simulink model "test5"  (R2015a)
settings: Solver=ode45  StartTime=0.0  StopTime=20  RelTol=1e-3
InitFcn:
  | %% DSPBuilder Start
  | alt_dspbuilder_update_model(bdroot)
  | %% DSPBuilder End
libraries: allblocks_alteradspbuilder2 x10
settings Model: Creator=ASUS  LastModifiedBy=ASUS

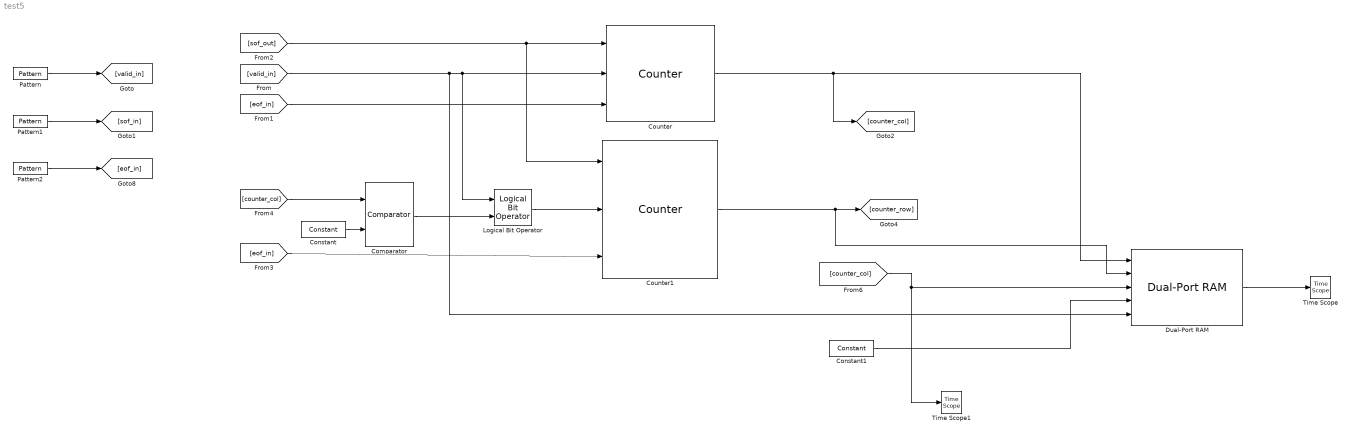
== system test5 ==
  Comparator : allblocks_alteradspbuilder2/Comparator  direction=a == b  pipeline_display=0  allowFloatingPointOverride=on  logOutputs=off  logFile=C:\Users\ASUS\Desktop\sift_fpga_final\Octave_2\tb_test5\test5_Comparator.fixedpointlog
  Constant : allblocks_alteradspbuilder2/Constant  mask_cst=3  BusType=Unsigned Integer  bwl=3  bwr=0  roundMode=Truncate  satMode=Wrap  SpecifyClock=off  allowFloatingPointOverride=on  logOutputs=off  logFile=C:\Users\ASUS\Desktop\sift_fpga_final\Octave_2\tb_test5\test5_Constant.fixedpointlog
  Constant1 : allblocks_alteradspbuilder2/Constant  mask_cst=1  BusType=Unsigned Integer  bwl=1  bwr=0  roundMode=Truncate  satMode=Wrap  SpecifyClock=off  allowFloatingPointOverride=on  logOutputs=off  logFile=C:\Users\ASUS\Desktop\sift_fpga_final\Octave_2\tb_test5\test5_Constant1.fixedpointlog
  Counter : allblocks_alteradspbuilder2/Counter  BusType=Unsigned Integer  bwl=5  bwr=0  use_modulo=on  modulo=4  SpecifyClock=off  direction=Increment  use_sload=off  use_sset=on  svalue=1  use_clk_ena=off  use_ena=on  use_sclr=on  pipeline_display=1
  Counter1 : allblocks_alteradspbuilder2/Counter  BusType=Unsigned Integer  bwl=5  bwr=0  use_modulo=on  modulo=4  SpecifyClock=off  direction=Increment  use_sload=off  use_sset=on  svalue=0  use_clk_ena=off  use_ena=on  use_sclr=on  pipeline_display=1
  Dual-Port RAM : allblocks_alteradspbuilder2/Dual-Port RAM  numwords=16  BusType=Signed Integer  bwl=8  bwr=0  memory_type=M9K  ram_type=DualRAM  dont_care=on  initialization=From MATLAB array  init_file=input.hex  init_array=[0:1:15]  register_outputs=on  use_ena=on  ClockPhase=1  allowFloatingPointOverride=on  logOutputs=off  logFile=C:\Users\ASUS\Desktop\sift_fpga_final\Octave_2\tb_test5\test5_Dual-Port+RAM.fixedpointlog  pipeline_display=2
  Logical Bit Operator : allblocks_alteradspbuilder2/Logical Bit Operator  LogicalOperator=AND  user_inputs=2  pipeline_display=0
  Pattern : allblocks_alteradspbuilder2/Pattern  Sequence=11111111111111111111111111111111111111111111111111111111111111111111  SpecifyClock=off  use_ena=off  use_sclr=off
  Pattern1 : allblocks_alteradspbuilder2/Pattern  Sequence=100000000000000000000000000000000000000000000000000000000000000000000000  SpecifyClock=off  use_ena=off  use_sclr=off
  Pattern2 : allblocks_alteradspbuilder2/Pattern  Sequence=00000000000000000000000000000000000000000000000000000000000000000000001  SpecifyClock=off  use_ena=off  use_sclr=off
  Time Scope : TimeScope  DefaultConfigurationName=spbscopes.TimeScopeBlockCfg
  Time Scope1 : TimeScope  DefaultConfigurationName=spbscopes.TimeScopeBlockCfg
  wires:
  [sof_out] -> Counter/1, Counter1/1
  [eof_in] -> Counter1/3
  Logical Bit Operator/1 -> Counter1/2
  [counter_col] -> Comparator/1
  Pattern1/1 -> [sof_in]
  Constant/1 -> Comparator/2
  Comparator/1 -> Logical Bit Operator/2
  Pattern/1 -> [valid_in]
  Counter1/1 -> Dual-Port RAM/2, [counter_row]
  Counter/1 -> [counter_col], Dual-Port RAM/1
  [valid_in] -> Dual-Port RAM/5, Counter/2, Logical Bit Operator/1
  Pattern2/1 -> [eof_in]
  [eof_in] -> Counter/3
  Dual-Port RAM/1 -> Time Scope/1
  Constant1/1 -> Dual-Port RAM/4
  [counter_col] -> Dual-Port RAM/3, Time Scope1/1
